simulink model "hybrid_photovoltaic_wind_power_sysytem_grid"  (R2024b)
settings: Solver=ode45  StartTime=0.0  StopTime=1  RelTol=1e-3  EnableMultiTasking=on
undefined symbols (not defined in the file): DiscIntNeverNeededParam, find_system
libraries: powerlib_extras x39, spsThreePhaseVIMeasurementLib x12, spsSeriesRLCBranchLib x5, spsDiodeLib x4, spsUniversalBridgeLib x4, simulink_extras x4, spsThreePhaseBreakerLib x3, spsLoadFlowBusLib x3, spsVoltageMeasurementLib x2, slpidlib x2, spsThreePhaseSeriesRLCLoadLib x2, spsThreePhaseTransformerInductanceMatrixTypeTwoWindingsLib x2
(part 1 of 4)
settings Model: Creator=venkat  LastModifiedBy=vinay
settings SolverCC: AlgebraicLoopSolver=TrustRegion
settings DataIOCC: LimitDataPoints=on  SaveFormat=Array  SignalLoggingSaveFormat=ModelDataLogs  ReturnWorkspaceOutputs=off
settings OptimizationCC: ExpressionDepthLimit=2147483647  LifeSpan=inf
settings DebuggingCC: UnderspecifiedInitializationDetection=Classic  MergeDetectMultiDrivingBlocksExec=none  SolverPrmCheckMsg=warning  FcnCallInpInsideContextMsg=warning  UnconnectedInputMsg=warning  UnconnectedOutputMsg=warning  UnconnectedLineMsg=warning  StateNameClashWarn=warning  SFUnexpectedBacktrackingDiag=warning  SFNoUnconditionalDefaultTransitionDiag=warning  SFExecutionAtInitializationDiag=none  ArithmeticOperatorsInVariantConditions=warning
settings HardwareCC: ProdBitPerPointer=32  ProdBitPerSizeT=32  ProdBitPerPtrDiffT=32  ProdLargestAtomicFloat=None  ProdIntDivRoundTo=Undefined  ProdEndianess=Unspecified  ProdWordSize=32  ProdHWDeviceType=32-bit Generic
settings ModelReferenceCC: EnableRefExpFcnMdlSchedulingChecks=on  PropagateSignalLabelsOutOfModel=off
settings SFSimCC: SimUseLocalCustomCode=off  CustomCodeUndefinedFunction=UseInterfaceOnly
settings RTWCC: RTWUseLocalCustomCode=off  GPUComputeCapability=3.5  DLArmComputeVersion=19.05
settings CodeAppCC: StateflowObjectComments=on
settings GRTTargetCC: TargetLangStandard=C89/C90 (ANSI)  CombineOutputUpdateFcns=off  GRTInterface=on
settings ConfigComp: CovMetricSettings=dw  CovSaveCumulativeToWorkspaceVar=on  CovSaveSingleToWorkspaceVar=on  CovExternalEMLEnable=off
settings SimscapeCC: SimscapeNormalizeSystem=off

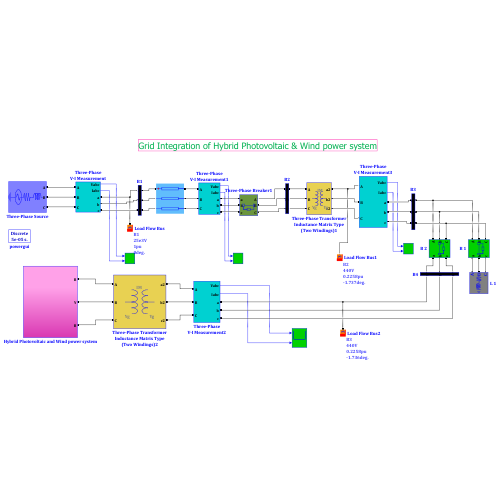
[thumbnail: Simulink's stored preview of the top-level diagram]
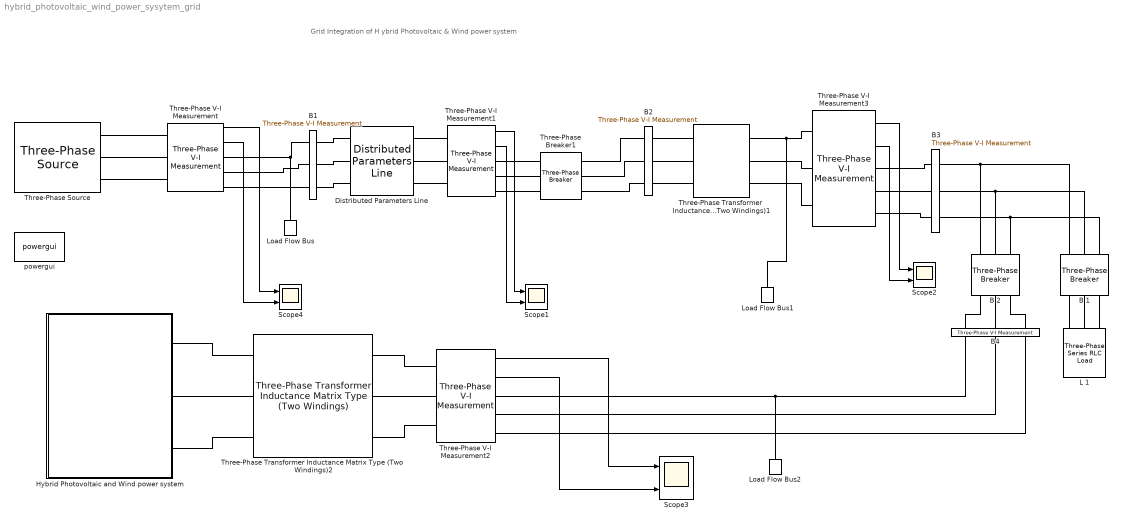
== system hybrid_photovoltaic_wind_power_sysytem_grid ==
  note: Grid Integration of H ybrid Photovoltaic & Wind power system
  B 1 : spsThreePhaseBreakerLib/Three-Phase Breaker  InitialState=closed  SwitchA=off  SwitchB=off  SwitchC=off  SwitchTimes="[0.02  0.4]"  External=off  BreakerResistance=0.001  SnubberResistance=1e6  SnubberCapacitance=inf  Measurements=None
  B 2 : spsThreePhaseBreakerLib/Three-Phase Breaker  InitialState=closed  SwitchA=off  SwitchB=off  SwitchC=off  SwitchTimes=[0.001 0.3]  External=off  BreakerResistance=0.001  SnubberResistance=1e6  SnubberCapacitance=inf  Measurements=None
  B1 : spsThreePhaseVIMeasurementLib/Three-Phase V-I Measurement  VoltageMeasurement=phase-to-ground  SetLabelV=on  LabelV=Vabc_B1  Vpu=off  VpuLL=off  CurrentMeasurement=no  SetLabelI=off  LabelI=A1  Ipu=off  Pbase=100e6  Vbase=25e3  OutputType=Magnitude  PhasorSimulation=off  PSBequivalent=0
  B2 : spsThreePhaseVIMeasurementLib/Three-Phase V-I Measurement  VoltageMeasurement=phase-to-ground  SetLabelV=on  LabelV=Vabc_B2  Vpu=off  VpuLL=off  CurrentMeasurement=yes  SetLabelI=on  LabelI=A2  Ipu=off  Pbase=100e6  Vbase=440  OutputType=Magnitude  PhasorSimulation=off  PSBequivalent=0
  B3 : spsThreePhaseVIMeasurementLib/Three-Phase V-I Measurement  VoltageMeasurement=phase-to-ground  SetLabelV=on  LabelV=Vabc_B3  Vpu=off  VpuLL=off  CurrentMeasurement=yes  SetLabelI=on  LabelI=A1  Ipu=off  Pbase=100e6  Vbase=440  OutputType=Magnitude  PhasorSimulation=off  PSBequivalent=0
  B4 : spsThreePhaseVIMeasurementLib/Three-Phase V-I Measurement  VoltageMeasurement=phase-to-phase  SetLabelV=on  LabelV=Vabc_B4  Vpu=off  VpuLL=off  CurrentMeasurement=yes  SetLabelI=on  LabelI=Iabc_B4  Ipu=off  Pbase=100e6  Vbase=440  OutputType=Magnitude  PhasorSimulation=off  PSBequivalent=0
  Distributed Parameters Line : spsDistributedParametersLineLib/Distributed Parameters Line  Phases=3  Length=100  Frequency=50  Resistance=[0.01273 0.3864]  Inductance="[0.9337e-3  4.1264e-3]"  Capacitance=[12.74e-9 7.751e-9]  x1=[-0.0006 7.90669957622914e-08 8343.04989423718 -24001.8540044251;-0.00055 7.82728037889709e-08 8719.02536979415 -23867.8460232251;-0.0005 7.74592991725365e-08 9092.84955630671 -23727.949008161;-0.00045 7.66266826330796e-08 9464.43021825048 -23582.1974767281;-0.0004 7.57751596062727e-08 9833.67567365721 -23430.6273909358;-0.00035 7.4904940192681e-08 10200.4948167359 -23273.2761484348;-0.0003 7.40162391059235e-08 10564.7971403519 -23110.1825732897;-0.00025 7.31092756196953e-08 10926.4927583579 -22941.3869063997;-0.0002 7.21842735136655e-08 11285.4924277724 -22766.9307955699;-0.00015 7.12414610182627e-08 11641.7075707988 -22586.8572852351;-0.0001 7.02810707583625e-08 11995.0502966807 -22401.2108058397;-5e-05 6.9303339695891e-08 12345.4334233877 -22210.0371628744]  x2=[-0.0006 3.59900680263241e-07 8376.65197170131 -24147.4259529429;-0.00055 3.57111090981103e-07 8754.90984663917 -24012.8722144004;-0.0005 3.54233389880834e-07 9131.0075785749 -23872.3936589513;-0.00045 3.51268286992119e-07 9504.85237102082 -23726.0249475771;-0.0004 3.4821651390973e-07 9876.35198336835 -23573.8021945673;-0.00035 3.45078823613009e-07 10245.414753647 -23415.7629586084;-0.0003 3.41855990280087e-07 10611.9496211406 -23251.946233517;-0.00025 3.38548809096864e-07 10975.8661488553 -23082.3924386188;-0.0002 3.35158096060811e-07 11337.0745458331 -22907.1434087756;-0.00015 3.31684687779633e-07 11695.485689307 -22726.2423840633;-0.0001 3.2812944126485e-07 12051.0111466903 -22539.7339991027;-5e-05 3.24493233720341e-07 12403.5631973964 -22347.6642720472]  x3=[-0.0006 1.55337357382061e-09 21.0108746560212 -91.3718539054767;-0.00055 1.57888274892892e-09 22.4434892992346 -91.0305571114422;-0.0005 1.60400235834426e-09 23.8705663472925 -90.6667998895599;-0.00045 1.62872620417889e-09 25.2917536902872 -90.2806719914813;-0.0004 1.65304818619379e-09 26.7067006715075 -89.8722686884876;-0.00035 1.67696230330383e-09 28.115058173958 -89.4416907479825;-0.0003 1.70046265505846e-09 29.5164787064987 -88.9890444086301;-0.00025 1.72354344309752e-09 30.9106164895831 -88.5144413541416;-0.0002 1.74619897258194e-09 32.2971275405743 -88.017998685719;-0.00015 1.7684236535988e-09 33.675669758617 -87.4998388931622;-0.0001 1.79021200254063e-09 35.0459030090467 -86.9600898246467;-5e-05 1.81155864345835e-09 36.4074892073121 -86.3988846551788]  x4=[-0.0006 -9.48429281222997e-10 30.9094555729155 -89.1998043499292;-0.00055 -9.77841104130026e-10 32.3067319811332 -88.7032953647736;-0.0005 -1.00701165937636e-09 33.6960371866506 -88.1849001687826;-0.00045 -1.03593374956399e-09 35.0770283991967 -87.6447466682139;-0.0004 -1.06460023859991e-09 36.4493648798542 -87.0829681378614;-0.00035 -1.09300405345692e-09 37.8127080251312 -86.4997031881712;-0.0003 -1.12113818591871e-09 39.1667214505066 -85.8950957310422;-0.00025 -1.14899569430908e-09 40.5110710734284 -85.2692949443175;-0.0002 -1.17656970520466e-09 41.845425195743 -84.6224552349772;-0.00015 -1.20385341513088e-09 43.169454585537 -83.9547362010405;-0.0001 -1.23084009224056e-09 44.4828325583705 -83.266302592188;-5e-05 -1.25752307797493e-09 45.7852350578811 -82.5573242691113]  x5=0.000565541566995743  V1=ones(3,3)  V2=ones(3,3)  I1=ones(3,3)  I2=ones(3,3)  nHarmo=1  Measurements=None  Decoupling=off  VsMag0=0  VrMag0=0  VsAngle0=0  VrAngle0=0  IsMag0=0  IrMag0=0  IsAngle0=0  IrAngle0=0
  Hybrid Photovoltaic and Wind power system : Subsystem
  L 1 : spsThreePhaseSeriesRLCLoadLib/Three-Phase Series RLC Load  LConnTagsString=A|B|C  Configuration=Y (grounded)  NominalVoltage=254.04  Vabc=[1e3 1e3 1e3]  Vabcp=[1e3 1e3 1e3]  NominalFrequency=50  UnbalancedPower=off  ActivePower=50e3  InductivePower=100  CapacitivePower=0  Pabc=[10e3 9e3 11e3]  QLabc=[100 90 110]  QCabc=[100 90 110]  Pabcp=[10e3 9e3 11e3]  QLabcp=[100 90 110]  QCabcp=[100 90 110]  Measurements=None  LoadType=constant Z
  Load Flow Bus : spsLoadFlowBusLib/Load Flow Bus  LConnTagsString=a  Phases=single  Connectors=on one side  ID=B1  Vbase=25e3  Vref=1  Vangle=0  VLF=1  VLFb=1  VLFc=1  angleLF=0  angleLFb=0  angleLFc=0
      settings: AttributesFormatString=%<ID>\n%<Vbase>V\n%<VLF>pu\n%<angleLF>deg.
  Load Flow Bus1 : spsLoadFlowBusLib/Load Flow Bus  LConnTagsString=a  Phases=single  Connectors=on one side  ID=B2  Vbase=440  Vref=1  Vangle=0  VLF=0.2258  VLFb=1  VLFc=1  angleLF=-1.737  angleLFb=0  angleLFc=0
      settings: AttributesFormatString=%<ID>\n%<Vbase>V\n%<VLF>pu\n%<angleLF>deg.
  Load Flow Bus2 : spsLoadFlowBusLib/Load Flow Bus  LConnTagsString=a  Phases=single  Connectors=on one side  ID=B3  Vbase=440  Vref=1  Vangle=0  VLF=0.2258  VLFb=1  VLFc=1  angleLF=-1.736  angleLFb=0  angleLFc=0
      settings: AttributesFormatString=%<ID>\n%<Vbase>V\n%<VLF>pu\n%<angleLF>deg.
  Scope{1..4} (4 alike) : Scope  NumInputPorts=2
  Three-Phase V-I Measurement{,1..3} (4 alike) : spsThreePhaseVIMeasurementLib/Three-Phase V-I Measurement  VoltageMeasurement=phase-to-ground  SetLabelV=off  LabelV=Vabc  Vpu=off  VpuLL=off  CurrentMeasurement=yes  SetLabelI=off  LabelI=Iabc  Ipu=off  Pbase=100e6  Vbase=500e3  OutputType=Complex  PhasorSimulation=off  PSBequivalent=0
  Three-Phase Breaker1 : spsThreePhaseBreakerLib/Three-Phase Breaker  InitialState=closed  SwitchA=off  SwitchB=off  SwitchC=off  SwitchTimes="[1/50  20/50]"  External=off  BreakerResistance=0.001  SnubberResistance=1e6  SnubberCapacitance=inf  Measurements=None
  Three-Phase Source : spsThreePhaseSourceLib/Three-Phase Source  InternalConnection=Yg  VoltagePhases=off  Voltage=(25000)*1.00008  PhaseAngle=0.13223  Voltage_phases=[25e3 25e3 25e3]/sqrt(3)  PhaseAngles_phases=[0 -120 +120]  Frequency=50  NonIdealSource=on  SpecifyImpedance=on  Resistance=0.8929  Inductance=16.58e-3  ShortCircuitLevel=100e6  BaseVoltage=63510.4  XRratio=7  BusType=swing  Pref=0  Qref=0  Prefabc=[10e3, 10e3, 10e3]  Qrefabc=[0, 0, 0]  Qmin=-inf  Qmax=inf
  Three-Phase Transformer Inductance Matrix Type (Two Windings)1 : spsThreePhaseTransformerInductanceMatrixTypeTwoWindingsLib/Three-Phase Transformer Inductance Matrix Type (Two Windings)  CoreType=Three-limb or five-limb core  Winding1Connection=Yg  Winding2Connection=Yg  AutoTransformer=off  Measurements=None  NominalPower=[100e3 50]  VLLnom=[63510.4 254.03]  WindingResistances=[0.01 0.01]  NoLoadIexcPos=2  NoLoadPlossPos=1000  ShortCircuitReactancePos=0.06  ShortCircuitReactancePosAuto=0.06  NoLoadIexcZero=100  NoLoadPlossZero=1500  ShortCircuitReactanceZero=0.03  ShortCircuitReactanceZeroAuto=0.03
  Three-Phase Transformer Inductance Matrix Type (Two Windings)2 : spsThreePhaseTransformerInductanceMatrixTypeTwoWindingsLib/Three-Phase Transformer Inductance Matrix Type (Two Windings)  CoreType=Three-limb or five-limb core  Winding1Connection=Yg  Winding2Connection=Yg  AutoTransformer=off  Measurements=None  NominalPower=[100e3 50]  VLLnom=[254.03 254.03]  WindingResistances=[0.01 0.01]  NoLoadIexcPos=2  NoLoadPlossPos=1000  ShortCircuitReactancePos=0.06  ShortCircuitReactancePosAuto=0.06  NoLoadIexcZero=100  NoLoadPlossZero=1500  ShortCircuitReactanceZero=0.03  ShortCircuitReactanceZeroAuto=0.03
  powergui : spspowerguiLib/powergui  Priority=1  SimulationMode=Discrete  SampleTime=50e-6  frequency=60  Iterations=50  frequencyindice=0  Pbase=100e6  ErrMax=0.0001  UnitsV=kV  UnitsW=MW  buscounter=0  FunctionMessages=off  echomessages=off  EnableUseOfTLC=off  CurrentSourceSwitches=off  DisableSnubberDevices=off  DisableRonSwitches=off  DisableVfSwitches=off  DisplayEquations=off  AutomaticDiscreteSolvers=off  SolverType=Tustin  Interpol=off  ExternalGateDelay=off  methode=off  Ts=100  x0status=blocks  SPID=off  SwTol=0  HookPort=off  NonlinearTolerance=1e-4  nMaxIteration=100  ContinueOnMaxIteration=off  RestoreLinks=warning  ResistiveCurrentMeasurement=off  Frange=[0:2:500]  Ylog=off  Xlog=on  ShowGrid=off  save=off  variable=ZData  structure=MLFCDSTAT  ZoomFFT=off  StartTime=0.8  cycles=10  DisplayStyle=1  fundamental=50  FreqAxis=on  MaxFrequency=50000  frequencyindicesteady=1  RmsSteady=1  display=off
  wires:
  Three-Phase V-I Measurement1/1 -> Scope1/1
  Three-Phase V-I Measurement1/2 -> Scope1/2
  Three-Phase V-I Measurement/1 -> Scope4/1
  Three-Phase V-I Measurement/2 -> Scope4/2
  Three-Phase V-I Measurement2/1 -> Scope3/1
  Three-Phase V-I Measurement2/2 -> Scope3/2
  Three-Phase V-I Measurement3/1 -> Scope2/1
  Three-Phase V-I Measurement3/2 -> Scope2/2
  connections:
  Three-Phase V-I Measurement/LConn3 -- Three-Phase Source/RConn3
  Three-Phase V-I Measurement/LConn2 -- Three-Phase Source/RConn2
  Three-Phase V-I Measurement/LConn1 -- Three-Phase Source/RConn1
  Three-Phase V-I Measurement/RConn3 -- B1/RConn3
  Three-Phase V-I Measurement/RConn2 -- B1/RConn2
  Three-Phase V-I Measurement/RConn1 -- Load Flow Bus/LConn1 -- B1/RConn1
  Distributed Parameters Line/LConn3 -- B1/LConn3
  Distributed Parameters Line/LConn2 -- B1/LConn2
  Distributed Parameters Line/LConn1 -- B1/LConn1
  Three-Phase V-I Measurement1/LConn3 -- Distributed Parameters Line/RConn3
  Three-Phase V-I Measurement1/LConn2 -- Distributed Parameters Line/RConn2
  Three-Phase V-I Measurement1/LConn1 -- Distributed Parameters Line/RConn1
  Three-Phase Transformer Inductance Matrix Type (Two Windings)1/LConn3 -- B2/LConn3
  Three-Phase Transformer Inductance Matrix Type (Two Windings)1/LConn2 -- B2/LConn2
  Three-Phase Transformer Inductance Matrix Type (Two Windings)1/LConn1 -- B2/LConn1
  Three-Phase V-I Measurement3/LConn3 -- Three-Phase Transformer Inductance Matrix Type (Two Windings)1/RConn3
  Three-Phase V-I Measurement3/LConn2 -- Three-Phase Transformer Inductance Matrix Type (Two Windings)1/RConn2
  Three-Phase V-I Measurement3/LConn1 -- Three-Phase Transformer Inductance Matrix Type (Two Windings)1/RConn1 -- Load Flow Bus1/LConn1
  Three-Phase V-I Measurement3/RConn1 -- B3/RConn1
  Three-Phase V-I Measurement3/RConn2 -- B3/RConn2
  Three-Phase V-I Measurement3/RConn3 -- B3/RConn3
  Three-Phase Breaker1/RConn1 -- Three-Phase V-I Measurement1/RConn1
  Three-Phase Breaker1/RConn2 -- Three-Phase V-I Measurement1/RConn2
  Three-Phase Breaker1/RConn3 -- Three-Phase V-I Measurement1/RConn3
  Three-Phase Breaker1/LConn1 -- B2/RConn1
  Three-Phase Breaker1/LConn2 -- B2/RConn2
  Three-Phase Breaker1/LConn3 -- B2/RConn3
  Three-Phase Transformer Inductance Matrix Type (Two Windings)2/RConn1 -- Three-Phase V-I Measurement2/LConn1
  Three-Phase Transformer Inductance Matrix Type (Two Windings)2/RConn2 -- Three-Phase V-I Measurement2/LConn2
  Three-Phase Transformer Inductance Matrix Type (Two Windings)2/RConn3 -- Three-Phase V-I Measurement2/LConn3
  B4/LConn1 -- B 2/RConn1
  B4/LConn2 -- B 2/RConn2
  B4/LConn3 -- B 2/RConn3
  B4/RConn3 -- Three-Phase V-I Measurement2/RConn3
  B4/RConn2 -- Three-Phase V-I Measurement2/RConn2
  Three-Phase V-I Measurement2/RConn1 -- B4/RConn1 -- Load Flow Bus2/LConn1
  B 1/LConn1 -- B3/LConn1 -- B 2/LConn1
  B 1/LConn2 -- B 2/LConn2 -- B3/LConn2
  L 1/LConn1 -- B 1/RConn1
  B 1/RConn2 -- L 1/LConn2
  L 1/LConn3 -- B 1/RConn3
  Hybrid Photovoltaic and Wind power system/RConn1 -- Three-Phase Transformer Inductance Matrix Type (Two Windings)2/LConn1
  Hybrid Photovoltaic and Wind power system/RConn2 -- Three-Phase Transformer Inductance Matrix Type (Two Windings)2/LConn2
  Hybrid Photovoltaic and Wind power system/RConn3 -- Three-Phase Transformer Inductance Matrix Type (Two Windings)2/LConn3
  B 1/LConn3 -- B 2/LConn3 -- B3/LConn3

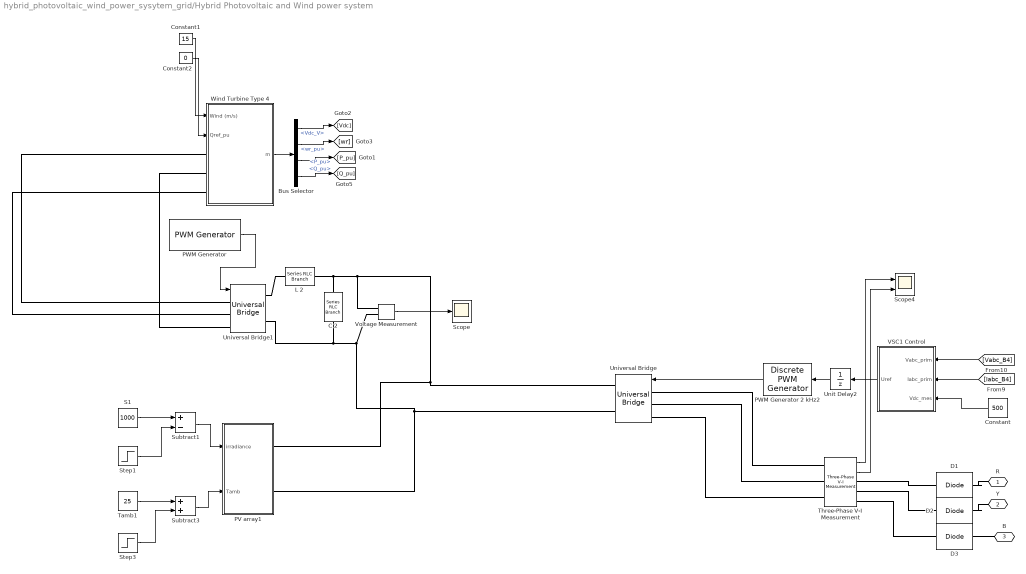
== system hybrid_photovoltaic_wind_power_sysytem_grid/Hybrid Photovoltaic and Wind power system ==
  Bus Selector : BusSelector  OutputSignals=Vdc_V,wr_pu,PQ_pu.P_pu,PQ_pu.Q_pu
  C 2 : spsSeriesRLCBranchLib/Series RLC Branch  LConnTagsString=__new0  RConnTagsString=__new0  BranchType=C  Resistance=1  Inductance=1e-4  SetiL0=off  InitialCurrent=0  Capacitance=3e-4  Setx0=off  InitialVoltage=0  Measurements=None
  Constant : Constant  Value=500
  Constant1 : Constant  Value=15
  Constant2 : Constant  Value=0
  D1 : spsDiodeLib/Diode  Ron=0.001  Lon=0  Vf=0.1  IC=0  UseSnubber=off  Rs=50000  Cs=250e-12  Measurements=off
  D2 : spsDiodeLib/Diode  Ron=0.001  Lon=0  Vf=0.1  IC=0  UseSnubber=off  Rs=50000  Cs=250e-12  Measurements=off
  D3 : spsDiodeLib/Diode  Ron=0.001  Lon=0  Vf=0.1  IC=0  UseSnubber=off  Rs=50000  Cs=250e-12  Measurements=off
  L 2 : spsSeriesRLCBranchLib/Series RLC Branch  LConnTagsString=__new0  RConnTagsString=__new0  BranchType=L  Resistance=1  Inductance=3e-2  SetiL0=off  InitialCurrent=0  Capacitance=1e-6  Setx0=off  InitialVoltage=0  Measurements=None
  PV array1 : Subsystem
  PWM Generator : powerlib_extras/Control  Blocks/PWM Generator  GeneratorMode="3-arm  bridge (6 pulses)"  Fc=1080  Internal=on  mIndex=0.4  Freq=50  Phase=0
  PWM Generator 2 kHz2 : powerlib_extras/Discrete  Control Blocks/Discrete PWM Generator  GeneratorMode="3-arm  bridge (6 pulses)"  Fc=33*50  Ts=1  Internal=off  mIndex=0.4  Freq=60  Phase=0
  S1 : Constant  Value=1000
  Scope : Scope
  Scope4 : Scope  NumInputPorts=2
  Step1 : Step  Time=3  After=200  SampleTime=0
  Step3 : Step  Time=2  After=5  SampleTime=0
  Subtract1 : Sum  Inputs=+-
  Subtract3 : Sum
  Tamb1 : Constant  Value=25
  Three-Phase V-I Measurement : spsThreePhaseVIMeasurementLib/Three-Phase V-I Measurement  VoltageMeasurement=phase-to-ground  SetLabelV=off  LabelV=Vabc  Vpu=off  VpuLL=off  CurrentMeasurement=yes  SetLabelI=off  LabelI=Iabc  Ipu=off  Pbase=100e6  Vbase=500e3  OutputType=Complex  PhasorSimulation=off  PSBequivalent=0
  Unit Delay2 : UnitDelay  HasFrameUpgradeWarning=on
  Universal Bridge : spsUniversalBridgeLib/Universal Bridge  Arms=3  SnubberResistance=1e5  SnubberCapacitance=inf  Device=MOSFET / Diodes  Ron=1e-3  Lon=0  ForwardVoltages="[  0  0  ]"  ForwardVoltage=0  GTOparameters=[ 10e-6 , 20e-6 ]  IGBTparameters=[ 1e-6 , 2e-6 ]  Measurements=None  Measurements_2=None  converterType=Rectifier
  Universal Bridge1 : spsUniversalBridgeLib/Universal Bridge  Arms=3  SnubberResistance=1e5  SnubberCapacitance=inf  Device=IGBT / Diodes  Ron=1e-3  Lon=0  ForwardVoltages="[  0  0  ]"  ForwardVoltage=0  GTOparameters=[ 10e-6 , 20e-6 ]  IGBTparameters=[ 1e-6 , 2e-6 ]  Measurements=None  Measurements_2=None  converterType=Rectifier
  VSC1 Control : Subsystem  mask(VSC Main Controller){nom=[ 50e3  50 ], Vnom=[ 6350.9 254.03 ], Vnom_dc=500, RLxfo=[0.008  0.04 ], RLchoke=[2e-3*(2*pi*60)/50   2e-3], K_VDCreg=[7  800], K_Ireg=[0.3 20]*1.5, Ts=1}
      mask prompts: nom "Nominal power and frequency [ Pnom(VA)  Fnom(Hz) ]:"; Vnom "Nominal primary and secondary voltages (Vrms LL) [ Vnom_prim   Vnom_sec ]:"; Vnom_dc "Nominal DC bus voltage (V):"; RLxfo "Total transformer leakage impedance (pu/Pnom) [ Rxfo  Lxf ]"; RLchoke "Choke impedance [ R(ohm) L(H) ]"; K_VDCreg "VDC regultator gains [ Kp  Ki ]:"; K_Ireg "Current regulator gains [ Kp  Ki ]:"; Ts "Sample time"
      mask init:
      | Pnom=nom(1);
      | Fnom=nom(2);
      | Vnom_prim=Vnom(1);
      | Vnom_sec=Vnom(2);
      | Zbase=Vnom_sec^2/Pnom;
      | Rtot_pu=RLxfo(1) + RLchoke(1)/Zbase;
      | Ltot_pu=RLxfo(2) + RLchoke(2)/(Zbase/(2*pi*Fnom));
      | Kp_VDCreg=K_VDCreg(1);
      | Ki_VDCreg=K_VDCreg(2);
      | Kp_Ireg=K_Ireg(1);
      | Ki_Ireg=K_Ireg(2);
      | Vdc_ref=Vnom_dc;
      | % Used to determine initial value of Boost Control (MPPT)
      | assignin('base','Vdc_ref_Inv',Vdc_ref);
  Voltage Measurement : spsVoltageMeasurementLib/Voltage Measurement  PhasorSimulation=off  OutputType=Complex  PSBequivalent=0
  Wind Turbine Type 4 : Subsystem  LoadFcn=%find_system(gcs,'FollowLinks', 'on', 'LookUnderMasks', 'all');  mask(Wind Turbine: Model 7){Nb_wt=1, ShowParameters=Control parameters for 1 wind turbine, nom=[1500/0.9 440 50], Reactances=[ 1.305, 0.296, 0.252, 0.474,  0.243,  0.18 ], Time_constants=[  4.49  0.0681  0.0513  ], Resistance=0.006, mec=[0.62 0.01 1], init=[ 0  0  0  0  0  0  0  0  1 ], Vnom=575, Imax_grid_conv=1.1, RL_grid=[ 0.15 0.15/50], C_var_filter1=150e3, Vdc_nom=1100, C_DClink1=90000e-6, L_R_Boost=[0.0012     5e-3], Pmec1=2e6, wind_speed_CpMax=11, wind0=11, DisplayTurbChar=off, H_WT=4.32, Ksh=0.3, D_mutual=1.5, w_wt0=1, torque0=1, Kdc=[1.1   27.5], Ki_var_reg=0.05, Ki_volt_reg=2, Kgrid_side_cur_reg=[1  50], Kspeed=[5 1], Kboost_cur_reg=[0.025 100], Kp_pitch=15, Kcompensation=[1.5  6], Kfield=[10  20], pitch_max=27, pitch_rate=10, Ts=0.1}
      mask prompts: Nb_wt "Number of wind turbines:"; ShowParameters "Display:"; nom "Nom. power, L-L volt. and freq.: [Pn (VA), Vn (Vrms), fn (Hz)]"; Reactances "Reactances [Xd Xd' Xd'' Xq Xq'' Xl] (p.u.):"; Time_constants "Time constants [Tdo' Tdo'' Tq''] (s):"; Resistance "Resistance Rs (p.u.):"; mec "Inertia constant, friction factor, and pairs of poles: [ H(s)  F(p.u.)  p ]"; init "Initial conditions: [dw(%) th(deg) ia,ib,ic(pu) pha,phb,phc(deg) Vf(pu)]:"; Vnom "Grid-side converter nominal AC voltage (V):"; Imax_grid_conv "Grid-side converter maximum AC current (pu based on generator power and converter nominal AC voltage):"; RL_grid "Grid-side coupling inductor [ L(pu) R(pu),pu based on generator power and converter nominal AC voltage] :"; C_var_filter1 "Line filter capacitor (Q=50) (var):"; Vdc_nom "Nominal DC bus voltage (V)"; C_DClink1 "DC bus capacitor (F):"; L_R_Boost "Boost converter inductance [L(H) R(ohm)]:"; Pmec1 "Nominal mechanical output power (W):"; wind_speed_CpMax "Wind speed at nominal speed and at Cp max (must be between 6 m/s and 30 m/s) (m/s):"; wind0 "Initial wind speed (m/s):"; DisplayTurbChar "Display wind turbine power characteristics:"; H_WT "Wind turbine inertia constant H (s):"; Ksh "Shaft spring constant refer to high-speed shaft (pu of nominal mechanical torque/rad):"; D_mutual "Shaft mutual damping (pu of nominal mechanical torque/pu dw):"; w_wt0 "Turbine initial speed (pu of nominal speed):"; torque0 "Initial output torque (pu of nominal mechanical torque):"; Kdc "DC bus voltage regulator gains [Kp Ki]:"; Ki_var_reg "Grid-side converter var regulator gain [ Ki]:"; Ki_volt_reg "Grid-side converter voltage regulator gain [ Ki]:"; Kgrid_side_cur_reg "Grid-side converter current regulator gains [Kp Ki]:"; Kspeed "Speed regulator gains [Kp Ki]:"; Kboost_cur_reg "Boost inductor current regulator gains [Kp Ki]:"; Kp_pitch "Pitch controller gain [Kp]:"; Kcompensation "Pitch compensation gains [Kp Ki]:"; Kfield "Field excitation gains [Kp Ki]:"; pitch_max "Maximum pitch angle (deg):"; pitch_rate "Maximum rate of change of pitch angle (deg/s)"; Ts "Sample time (s):"
      mask help: This block implements a model of a variable speed pitch controlled wind turbine using a synchronous generator.
      mask init:
      | %Generator data
      | Pnom=nom(1)*Nb_wt;
      | Vnom_gen=nom(2);
      | Fnom=nom(3);
      | Xd=Reactances(1);
      | Xd1=Reactances(2);
      | Xd2=Reactances(3);
      | Xq=Reactances(4);
      | Xq2=Reactances(5);
      | Xl=Reactances(6);
      | Tdo1=Time_constants(1);
      | Tdo2=Time_constants(2);
      | Tq2=Time_constants(3);
      | H=mec(1);
      | F=mec(2);
      | p=mec(3);
      | 
      | % Converters data
      | L_RL=RL_grid(1);
      | R_RL=RL_grid(2);
      | L_Boost=L_R_Boost(1)/Nb_wt;
      | R_Boost=L_R_Boost(2)/Nb_wt;
      | Q_filter=50;
      | C_DClink=C_DClink1*Nb_wt;
      | C_var_filter=C_var_filter1*Nb_wt;
      | 
      | % Controller data
      | Freq_filter=10000;   %Hz
      | Zeta_filter=0.707;
      | Kp_dc=Kdc(1);
      | Ki_dc=Kdc(2);
      | Kp_grid_side_cur_reg=Kgrid_side_cur_reg(1);
      | Ki_grid_side_cur_reg=Kgrid_side_cur_reg(2);
      | Kp_speed=Kspeed(1);
      | Ki_speed=Kspeed(2);
      | Kp_boost_cur_reg=Kboost_cur_reg(1);
      | Ki_boost_cur_reg=Kboost_cur_reg(2);
      | Kp_compensation=Kcompensation(1);
      | Ki_compensation=Kcompensation(2);
      | Kp_field=Kfield(1);
      | Ki_field=Kfield(2);
      | Mod_index_max=1.1;
      | T_speed=5;      %Speed reference time constant (s)
      | Iq_ref_limit_time_constant=0.3; %(s)
      | Current_reg_output_limit=1.1;   %(pu)
      | Var_reg_output_hi_limit=1.1;    %(pu)
      | Var_reg_output_low_limit=0.9;   %(pu)
      | Pitch_time_constant=0.01;       %(s)
      | Vf_limit=10;    %Field voltage limit (pu)
      | Flux_meas_time_constant=1*(1/Fnom); %(s)
      | Freq_sawtooth=2000; %Hz, Boost converter
      | Freq_PWM=3000; %Hz, Inverter
      | Ts_snub=50e-6;  %Sample time to compute snubber resistance
      | 
      | 
      | % Turbine data
      | Pmec=Pmec1*Nb_wt;
      | c1 = 0.6450;
      | c2 = 116;
      | c3 = .4;
      | c4 = 5;
      | c5 = 21;
      | c6 = .00912;  % Set Pmin in stall condition (does not vary with wind_speed_Pmax)
      | c7 = .08;
      | c8 = .035;
      | theta=0;
      | CpMax=.5;
      | lambda_CpMax=9.9495;
      | 
      | c1_c8=[c1 c2 c3 c4 c5 c6 c7 c8];
      |   
      | 
      | %   Cp = c1*(c6*lambda + (-c4 - c3*(2.5 + theta) + c2*(1/(lambda + ...
      | %   c7*(2.5 + theta)) - c8/(1 + (2.5 + theta)^3)))/exp(c5*(1/(lambda + ...
      | %   c7*(2.5 + theta)) - c8/(1 + (2.5 + theta)^3))))
      | 
      | 
      |         %%%%%%%%%%%%%%%%%%%%%%%%%%%%%%%%%%%%%%%%%%%%%%%%%%%%%%%%%%%%%%%%%%%%%%%%%%%
      |         % Operation at Cp max
      |         %%%%%%%%%%%%%%%%%%%%%%%%%%%%%%%%%%%%%%%%%%%%%%%%%%%%%%%%%%%%%%%%%%%%%%%%%%%
      |         
      |         rated_omegar=1;
      |         omegar = rated_omegar;
      |         
      |         % Enforce boundaries on wind speed
      |         % A warning could be displayed
      |         if wind_speed_CpMax < 6
      |             wind_speed_CpMax=6;
      |             disp('Warning: Wind speed at nominal speed and at Cp max has been set to 6 m/s')
      |         end
      |         if wind_speed_CpMax > 30
      |             wind_speed_CpMax=30;
      |             disp('Warning: Wind speed at nominal speed and at Cp max has been set to 30 m/s')
      |         end
      | 
      |         K1=lambda_CpMax/omegar*wind_speed_CpMax;
      |         
      |         % Calculation of K2 needed to get P equal to the requested value at
      |         % Cp max for the requested wind speed
      |         
      |         Prated=Pmec;
      |         P_rated_omegar_theta_zero=0.75;
      |         
      |         K2 = P_rated_omegar_theta_zero*Prated/(wind_speed_CpMax^3*CpMax);
      |         
      |         K1_K2=[K1 K2];
      |         
      |         %%%%%%%%%%%%%%%%%%%%%%%%%%%%%%%%%%%%%%%%%%%%%%%%%%%%%%%%%%%%%%%%%%%%%%%%%%%
      |         % End of calculation for operation at Cp max
      |         %%%%%%%%%%%%%%%%%%%%%%%%%%%%%%%%%%%%%%%%%%%%%%%%%%%%%%%%%%%%%%%%%%%%%%%%%%%
      |         
      | 
      | %%%%%%%%%%%%%%%%%%%%%%%%%%%%%%%%%%%%%%%%%%%%%%%%%%%%%%%%%%%%%%%%%%%%%%%%%%%
      | % Plot turbine characteristics
      | %%%%%%%%%%%%%%%%%%%%%%%%%%%%%%%%%%%%%%%%%%%%%%%%%%%%%%%%%%%%%%%%%%%%%%%%%%% 
      | 
      | DisplayTurbChar=get_param(gcb,'DisplayTurbChar');
      | if strcmp(DisplayTurbChar,'on')
      |     vect_theta = 0:2:30;
      |     
      |     vect_lambda = 1:0.2:30;
      |     
      |     clear Cp;
      |     
      |     for i=1:length(vect_theta)
      |      for j=1:length(vect_lambda)
      |                 Cp(i,j) = c1*(c6*vect_lambda(j) + (-c4 - c3*(2.5 + vect_theta(i)) + c2*(1/(vect_lambda(j) + ...
      |                 c7*(2.5 + vect_theta(i))) - c8/(1 + (2.5 + vect_theta(i))^3)))/exp(c5*(1/(vect_lambda(j) + ...
      |                 c7*(2.5 + vect_theta(i))) - c8/(1 + (2.5 + vect_theta(i))^3))));
      |      end
      |     end
      | 
      |     figure(1);
      |     clf;
      |     hold on;
      | 
      |     plot(vect_lambda, Cp);
      |     axis([0, 25, 0, .6]);
      |     title('Wind Turbine Cp Characteristic (pitch angle increases by step of 2 deg.)');
      |     ylabel('Cp');
      |     set(gca,'ytick',[0 .1 .2 .3 .4 .5 .6]);
      |     xlabel('Lambda');
      |     grid on;
      |     text(10.1,0.51,'Pitch angle 0 degree');
      | 
      |     hold off
      |     
      |     % Plot of the wind turbine mechanical power output (pu) lambda and Cp
      |     % characteristics against wind speed (m/s) for a range of theta.
      |     
      |     wind_speed_range = [1,.2,30];
      |     vect_wind_speed = 1:0.2:30;
      |     
      |     clear lambda;
      |     clear Cp;
      |     clear P;
      | 
      |     for i=1:length(vect_theta)
      |         for j=1:length(vect_wind_speed)
      |             lambda(i,j) = K1*omegar/vect_wind_speed(j);
      |             Cp(i,j) = c1*(c6*lambda(i,j) + (-c4 - c3*(2.5 + vect_theta(i)) + c2*(1/(lambda(i,j) + ...
      |             c7*(2.5 + vect_theta(i))) - c8/(1 + (2.5 + vect_theta(i))^3)))/exp(c5*(1/(lambda(i,j) + ...
      |             c7*(2.5 + vect_theta(i))) - c8/(1 + (2.5 + vect_theta(i))^3))));
      |             P(i,j) = K2/Prated*vect_wind_speed(j)^3*Cp(i,j);
      |         end
      |     end
      |     
      |     
      |     figure(2);
      |     clf;
      |     hold on
      |     
      |     subplot(3,1,1);
      |     plot(vect_wind_speed, P);
      |     axis([0, 35, 0, 1.5]);
      |     title('Wind Turbine Characteristics (w = 1 pu, pitch angle increases by step of 2 deg.)');
      |     ylabel('P (pu)');
      |     set(gca,'ytick',0:.5:4);
      |     grid on;
      |     
      |     subplot(3,1,2);
      |     plot(vect_wind_speed, lambda);
      |     axis([0, 35, 0, 20]);
      |     ylabel('Lambda');
      |     grid on;
      |     
      |     subplot(3,1,3)
      |     plot(vect_wind_speed, Cp);
      |     axis([0, 35, 0, .6]);
      |     xlabel('Wind Speed (m/s)');
      |     ylabel('Cp');
      |     set(gca,'ytick',[0 .1 .2 .3 .4 .5 .6]);
      |     grid on;
      | 
      |     hold off
      |     set_param(gcb,'DisplayTurbChar','off')
      |     
      | end
      mask TypeOptions ShowParameters: Generator data for 1 wind turbine | Converters data for 1 wind turbine | Turbine data for 1 wind turbine | Drive train data for 1 wind turbine | Control parameters for 1 wind turbine
      mask Callback ShowParameters:
      | BlockName=getfullname(gcb);
      | %
      | Param_Show=get_param(BlockName,'ShowParameters');
      | Param_DisplayTurbChar=get_param(BlockName,'DisplayTurbChar');
      | 
      | p_mask{3}='off';p_mask{4}='off';p_mask{5}='off';
      | p_mask{6}='off';p_mask{7}='off';p_mask{8}='off';p_mask{9}='off';
      | p_mask{10}='off';p_mask{11}='off';p_mask{12}='off';p_mask{13}='off';
      | p_mask{14}='off';p_mask{15}='off';p_mask{16}='off';p_mask{17}='off';
      | p_mask{18}='off';p_mask{19}='off';p_mask{20}='off';p_mask{21}='off';
      | p_mask{22}='off';p_mask{23}='off';p_mask{24}='off';p_mask{25}='off';
      | p_mask{26}='off';p_mask{27}='off';p_mask{28}='off';p_mask{29}='off';
      | p_mask{30}='off';p_mask{31}='off';p_mask{32}='off';p_mask{33}='off';
      | p_mask{34}='off';p_mask{35}='off';
      | 
      | switch Param_Show
      | 	case 'Generator data for 1 wind turbine'
      | 		p_mask{3}='on';p_mask{4}='on';p_mask{5}='on';
      |         p_mask{6}='on';p_mask{7}='on';p_mask{8}='on';
      |     case 'Converters data for 1 wind turbine'
      | 		p_mask{9}='on';p_mask{10}='on';p_mask{11}='on';
      |         p_mask{12}='on';p_mask{13}='on';p_mask{14}='on';p_mask{15}='on';
      | 	case 'Turbine data for 1 wind turbine'
      | 		p_mask{16}='on';p_mask{17}='on';p_mask{18}='on';p_mask{19}='on';
      |     case 'Drive train data for 1 wind turbine'
      |         p_mask{20}='on';p_mask{21}='on';p_mask{22}='on';p_mask{23}='on';
      |         p_mask{24}='on';
      |     case 'Control parameters for 1 wind turbine'
      |         p_mask{25}='on';p_mask{26}='on';p_mask{27}='on';
      |         p_mask{28}='on';p_mask{29}='on';p_mask{30}='on';p_mask{31}='on';
      |         p_mask{32}='on';p_mask{33}='on';p_mask{34}='on';p_mask{35}='on';
      | end
      | 
      | ParVisible={'on','on',p_mask{3},p_mask{4},p_mask{5},p_mask{6},...
      |     p_mask{7},p_mask{8},p_mask{9},p_mask{10},p_mask{11},p_mask{12},...
      |     p_mask{13},p_mask{14},p_mask{15},p_mask{16},p_mask{17},p_mask{18},...
      |     p_mask{19},p_mask{20},p_mask{21},p_mask{22},p_mask{23},p_mask{24},...
      |     p_mask{25},p_mask{26},p_mask{27},p_mask{28},p_mask{29},p_mask{30},...
      |     p_mask{31},p_mask{32},p_mask{33},p_mask{34},p_mask{35},'on'};
      | %
      | set_param(BlockName,'MaskVisibilities',ParVisible);
      | set_param(BlockName,'DisplayTurbChar',Param_DisplayTurbChar);
      mask Display: disp(' ');
  R : PMIOPort  Side=Right
  Y : PMIOPort  Port=2  Side=Right
  B : PMIOPort  Port=3  Side=Right
  wires:
  [Vabc_B4] -> VSC1 Control/1(Vabc_prim)
  [Iabc_B4] -> VSC1 Control/2(Iabc_prim)
  PWM Generator 2 kHz2/1 -> Universal Bridge/1
  Constant/1 -> VSC1 Control/3(Vdc_mes)
  Three-Phase V-I Measurement/1 -> Scope4/1
  Three-Phase V-I Measurement/2 -> Scope4/2
  Unit Delay2/1 -> PWM Generator 2 kHz2/1
  VSC1 Control/1(Uref) -> Unit Delay2/1
  Voltage Measurement/1 -> Scope/1
  Subtract3/1 -> PV array1/2(Tamb)
  S1/1 -> Subtract1/1
  Subtract1/1 -> PV array1/1(irradiance)
  Step1/1 -> Subtract1/2
  Tamb1/1 -> Subtract3/1
  Step3/1 -> Subtract3/2
  Constant1/1 -> Wind Turbine Type 4/1("Wind (m/s) ")
  Wind Turbine Type 4/1(m) -> Bus Selector/1
  Constant2/1 -> Wind Turbine Type 4/2(Qref_pu)
  Bus Selector/1 -> [Vdc]  "<Vdc_V>"
  Bus Selector/2 -> [wr]  "<wr_pu>"
  Bus Selector/3 -> [P_pu]  "<P_pu>"
  Bus Selector/4 -> [Q_pu]  "<Q_pu>"
  PWM Generator/1 -> Universal Bridge1/1
  connections:
  Three-Phase V-I Measurement/LConn1 -- Universal Bridge/LConn1
  Three-Phase V-I Measurement/LConn2 -- Universal Bridge/LConn2
  Three-Phase V-I Measurement/RConn2 -- D2/LConn1
  D3/RConn1 -- B/RConn1
  D2/RConn1 -- Y/RConn1
  Three-Phase V-I Measurement/LConn3 -- Universal Bridge/LConn3
  Three-Phase V-I Measurement/RConn1 -- D1/LConn1
  D1/RConn1 -- R/RConn1
  Three-Phase V-I Measurement/RConn3 -- D3/LConn1
  Voltage Measurement/LConn1 -- PV array1/RConn1 -- Universal Bridge/RConn1 -- C 2/LConn1 -- L 2/RConn1
  PV array1/RConn2 -- Voltage Measurement/LConn2 -- Universal Bridge1/RConn2 -- C 2/RConn1 -- Universal Bridge/RConn2
  L 2/LConn1 -- Universal Bridge1/RConn1
  Wind Turbine Type 4/LConn3 -- Universal Bridge1/LConn2
  Wind Turbine Type 4/LConn1 -- Universal Bridge1/LConn1
  Wind Turbine Type 4/LConn2 -- Universal Bridge1/LConn3

== system hybrid_photovoltaic_wind_power_sysytem_grid/Hybrid Photovoltaic and Wind power system/PV array1 ==
  irradiance : Inport
  Tamb : Inport  Port=2
  4700uF : spsSeriesRLCBranchLib/Series RLC Branch  LConnTagsString=__new0  RConnTagsString=__new0  BranchType=C  Resistance=1  Inductance=5e-03  SetiL0=off  InitialCurrent=0  Capacitance=4700e-6  Setx0=off  InitialVoltage=0  Measurements=None
  CCS : spsControlledCurrentSourceLib/Controlled Current Source  Initialize=on  Source_Type=AC  Amplitude=0  Phase=0  Frequency=0  Measurements=None
  CM : spsCurrentMeasurementLib/Current Measurement  PhasorSimulation=off  OutputType=Complex  PSBequivalent=0
  Divide1 : Product  Inputs=**
  Im : Constant  Value=1.93
  Isc : Constant  Value=2.02
  Saturation : Saturate  UpperLimit=100  LowerLimit=0
  Saturation1 : Saturate  UpperLimit=4  LowerLimit=0
  Subsystem1 : Subsystem
  Tref : Constant  Value=55
  VM1 : spsVoltageMeasurementLib/Voltage Measurement  PhasorSimulation=off  OutputType=Complex  PSBequivalent=0
  Vm : Constant  Value=70.4
  Voc : Constant  Value=86.8
  + : PMIOPort  Tag=PMCPort  Side=Right
  - : PMIOPort  Tag=PMCPort  Port=2  Side=Right
  tag scope: Ipv1=global, Ppv1=global, Upv1=global
  wires:
  Saturation1/1 -> CCS/1
  CM/1 -> Divide1/2, [Ipv1]
  Divide1/1 -> [Ppv1]
  Subsystem1/2(Ipv) -> Saturation1/1
  Tref/1 -> Subsystem1/9(Tref)
  VM1/1 -> Divide1/1, [Upv1], Saturation/1
  Saturation/1 -> Subsystem1/1(Vpv)
  Tamb/1 -> Subsystem1/3(Tamb)
  irradiance/1 -> Subsystem1/2(S)
  Vm/1 -> Subsystem1/8(Vm)
  Voc/1 -> Subsystem1/6(Voc)
  Im/1 -> Subsystem1/7(Im)
  Isc/1 -> Subsystem1/4(Isc)
  Subsystem1/1(Out1) -> Subsystem1/5(In5)
  connections:
  4700uF/RConn1 -- VM1/LConn2 -- CCS/LConn1 -- -/RConn1
  4700uF/LConn1 -- VM1/LConn1 -- CM/RConn1 -- +/RConn1
  CCS/RConn1 -- CM/LConn1

== system hybrid_photovoltaic_wind_power_sysytem_grid/Hybrid Photovoltaic and Wind power system/VSC1 Control ==
  note: VSC Main Controller
  Vabc_prim : Inport  PortDimensions=3
  Iabc_prim : Inport  Port=2  PortDimensions=3
  Vdc_mes : Inport  Port=3  PortDimensions=1
  Current Regulator : Subsystem
  Gain : Gain  Gain=-1
  Iq_ref : Constant  Value=0
  Mux : Mux  Inputs=2
  PLL & Measurements : Subsystem
  Uabc_ref Generation max (m) = 1 : Subsystem
  VDC Regulator : Subsystem
  Vdc_ref1 : Constant  Value=Vdc_ref
  Uref : Outport
  wires:
  Vdc_ref1/1 -> VDC Regulator/2(Vdc_ref)
  Uabc_ref Generation max (m) = 1/1(Uabc_ref) -> Uref/1
  Iabc_prim/1 -> Gain/1
  Vabc_prim/1 -> PLL & Measurements/1(Vabc_prim)
  Vdc_mes/1 -> VDC Regulator/1(Vdc_mes)
  PLL & Measurements/2(VdVq_prim) -> Current Regulator/1(VdVq_mes)
  PLL & Measurements/3(IdIq_prim) -> Current Regulator/2(IdIq_mes)
  Mux/1 -> Current Regulator/3(IdIq_ref)
  Iq_ref/1 -> Mux/2
  Current Regulator/1(VdVq_conv) -> Uabc_ref Generation max (m) = 1/2(VdVq_conv)
  PLL & Measurements/1(wt) -> Uabc_ref Generation max (m) = 1/1(wt)
  VDC Regulator/1(Id_ref) -> Mux/1
  Gain/1 -> PLL & Measurements/2(Iabc_prim)

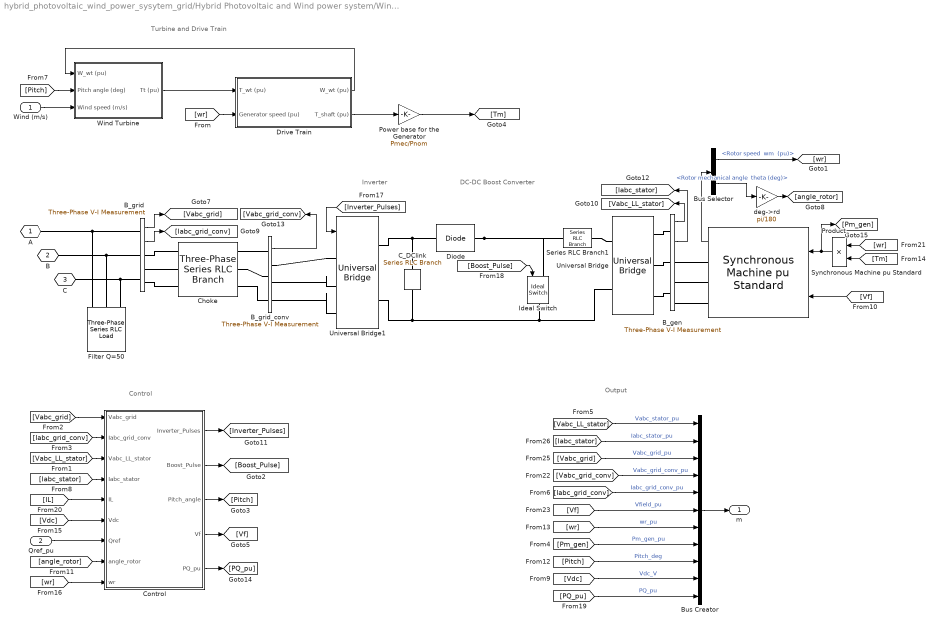
== system hybrid_photovoltaic_wind_power_sysytem_grid/Hybrid Photovoltaic and Wind power system/Wind Turbine Type 4 ==
  note: Turbine and Drive Train
  note: Control
  note: Inverter
  note: DC-DC Boost Converter
  note: Output
  "Wind (m/s) " : Inport
  Qref_pu : Inport  Port=2
  B_gen : spsThreePhaseVIMeasurementLib/Three-Phase V-I Measurement  VoltageMeasurement=phase-to-phase  SetLabelV=off  LabelV=Vabc  Vpu=on  VpuLL=off  CurrentMeasurement=yes  SetLabelI=off  LabelI=Iabc  Ipu=on  Pbase=Pnom  Vbase=Vnom_gen  OutputType=Complex  PhasorSimulation=off  PSBequivalent=0
  B_grid : spsThreePhaseVIMeasurementLib/Three-Phase V-I Measurement  VoltageMeasurement=phase-to-ground  SetLabelV=off  LabelV=Vabc  Vpu=on  VpuLL=off  CurrentMeasurement=yes  SetLabelI=off  LabelI=Iabc  Ipu=on  Pbase=Pnom  Vbase=Vnom  OutputType=Complex  PhasorSimulation=off  PSBequivalent=0
  B_grid_conv : spsThreePhaseVIMeasurementLib/Three-Phase V-I Measurement  VoltageMeasurement=phase-to-ground  SetLabelV=off  LabelV=Vabc  Vpu=on  VpuLL=off  CurrentMeasurement=no  SetLabelI=off  LabelI=Iabc  Ipu=on  Pbase=Pnom  Vbase=Vnom  OutputType=Complex  PhasorSimulation=off  PSBequivalent=0
  Bus Creator : BusCreator  Inputs=11
  Bus Selector : BusSelector  OutputSignals="Mechanical.Rotor speed  wm  (pu),Mechanical.Rotor mechanical angle  theta (deg)"
  C_DClink : spsSeriesRLCBranchLib/Series RLC Branch  LConnTagsString=__new0  RConnTagsString=__new0  BranchType=C  Resistance=1  Inductance=1e-3  SetiL0=off  InitialCurrent=0  Capacitance=C_DClink  Setx0=on  InitialVoltage=Vdc_nom  Measurements=Branch voltage
  "Choke " : spsThreePhaseSeriesRLCBranchLib/Three-Phase Series RLC Branch  LConnTagsString=A|B|C  RConnTagsString=A|B|C  BranchType=RL  Resistance=R_RL*Vnom^2/Pnom  Inductance=L_RL*Vnom^2/Pnom/(2*pi*Fnom)  Capacitance=[]  Measurements=None
  Control : Subsystem
  Diode : spsDiodeLib/Diode  Ron=1e-6/Nb_wt  Lon=0  Vf=0  IC=0  UseSnubber=off  Rs=inf  Cs=inf  Measurements=off
  Drive Train : Subsystem  mask(Wind Turbine shaft){H_WT=H_WT, Ksh=Ksh, D_mutual=D_mutual, wbase=2*pi*Fnom/p, w_wt0=w_wt0, torque0=torque0, Ts=Ts}
      mask prompts: H_WT "Wind turbine inertia constant H (s):"; Ksh "Shaft spring constant (pu of nominal mechanical torque/rad):"; D_mutual "Shaft mutual damping (pu of nominal mechanical torque/pu dw):"; wbase "Shaft base speed (rad/s):"; w_wt0 "Turbine initial speed (pu of base speed):"; torque0 "Initial output torque (pu of nominal mechanical torque):"; Ts "Sample time (s):"
      mask help:
      | This block implements a wind turbine drive train model. All shaft parameters are referred to high-speed shaft (generator shaft).
      |
      | The first input is the wind turbine torque in per unit (pu) based on the nominal power of the turbine and the base speed of the generator. The second input is the generator speed in pu based on the base speed of the generator.
      |
      | The outputs are:
      | 1- the transmitted torque of the shaft in pu based on the nominal power of the turbine and the base speed of the generator.
      | 2- the wind turbine speed in pu of the base speed of the generator.
  Filter Q=50 : spsThreePhaseSeriesRLCLoadLib/Three-Phase Series RLC Load  LConnTagsString=A|B|C  Configuration=Y (grounded)  NominalVoltage=Vnom  Vabc=[1e3 1e3 1e3]  Vabcp=[1e3 1e3 1e3]  NominalFrequency=Fnom  UnbalancedPower=off  ActivePower=C_var_filter/Q_filter  InductivePower=0  CapacitivePower=C_var_filter  Pabc=[10e3 9e3 11e3]  QLabc=[100 90 110]  QCabc=[100 90 110]  Pabcp=[10e3 9e3 11e3]  QLabcp=[100 90 110]  QCabcp=[100 90 110]  Measurements=None  LoadType=constant Z
  Ideal Switch : spsIdealSwitchLib/Ideal Switch  Ron=1e-6/Nb_wt  Lon=0  IC=0  Rs=1e5/Nb_wt  Cs=inf  Measurements=off
  Power base for the Generator : Gain  Gain=Pmec/Pnom  SaturateOnIntegerOverflow=on  OutDataTypeStr=Inherit: Same as input  ParamDataTypeStr=Inherit: Same as input
  Product : Product  RndMeth=Zero
  Series RLC Branch1 : spsSeriesRLCBranchLib/Series RLC Branch  LConnTagsString=__new0  RConnTagsString=__new0  BranchType=RL  Resistance=R_Boost  Inductance=L_Boost  SetiL0=off  InitialCurrent=0  Capacitance=1.0  Setx0=off  InitialVoltage=0  Measurements=Branch current
  Synchronous Machine pu Standard : spsSynchronousMachinepuStandardLib/Synchronous Machine pu Standard  PresetModel=No  MechanicalLoad=Mechanical power Pm  ShowDetailedParameters=on  RotorType=Salient-pole  Units=per unit standard parameters  MeasurementBus=off  NominalParameters="[ Pnom  Vnom_gen Fnom ]"  Reactances1=[ 1.81, 0.3, 0.23, 1.76, 0.65, 0.25, 0.15 ]  Reactances2="[ Xd, Xd1, Xd2, Xq,  Xq2,  Xl ]"  dAxisTimeConstants=Open-circuit  qAxisTimeConstants=Short-circuit  TimeConstants1="[ 4.4849  0.0681  0.1  ]"  TimeConstants2=[ 8.0, 0.03, 1.0, 0.07 ]  TimeConstants3="[  Tdo1  Tdo2  Tq2  ]"  TimeConstants4=[ 8.0, 0.03, 0.3371, 0.0295 ]  TimeConstants5=[ 1.01, 0.053, 0.1 ]  TimeConstants6=[ 1.3201, 0.023, 1.0, 0.07 ]  TimeConstants7="[  1.01  0.053  0.051266  ]"  TimeConstants8=[ 1.3201, 0.0231, 0.3371, 0.0295 ]  StatorResistance=Resistance  Mechanical=[ H F p]  PolePairs=1  InitialConditions=init  SetSaturation=off  Saturation=[0.6404,0.7127,0.8441,0.9214,0.9956,1.082,1.19,1.316,1.457;0.7,0.7698,0.8872,0.9466,0.9969,1.046,1.1,1.151,1.201]  LoadFlowParameters=[1 0 0 0 0]  TsPowergui=0  TsBlock=-1  IterativeModel=Trapezoidal non iterative  IterativeDiscreteModel=Trapezoidal non iterative  BusType=PV  Pref=0  Qref=0  Qmin=-inf  Qmax=inf  PLF=0  QLF=0
  Universal Bridge : spsUniversalBridgeLib/Universal Bridge  Arms=3  SnubberResistance=2*Ts_snub/(Pnom/(1000*2*pi*Fnom*Vnom_gen^2))  SnubberCapacitance=Pnom/(1000*2*pi*Fnom*Vnom_gen^2)  Device=Diodes  Ron=1e-6/Nb_wt  Lon=0  ForwardVoltages="[  0  0  ]"  ForwardVoltage=0  GTOparameters=[ 10e-6 , 20e-6 ]  IGBTparameters=[ 1e-6 , 2e-6 ]  Measurements=None  Measurements_2=None  converterType=Rectifier
  Universal Bridge1 : spsUniversalBridgeLib/Universal Bridge  Arms=3  SnubberResistance=1e6/Nb_wt  SnubberCapacitance=inf  Device=IGBT / Diodes  Ron=1e-6/Nb_wt  Lon=0  ForwardVoltages="[  0  0  ]"  ForwardVoltage=0  GTOparameters=[ 10e-6 , 20e-6 ]  IGBTparameters=[ 1e-6 , 2e-6 ]*0  Measurements=None  Measurements_2=None  converterType=Rectifier
  Wind Turbine : Subsystem  mask(Wind Turbine){Prated=Pmec, c1_c8=c1_c8, K1_K2=K1_K2, wind0=wind0, Ts=Ts}
      mask prompts: Prated "Nominal mechanical output power (W):"; c1_c8 "Coefficients [c1 ... c8]"; K1_K2 "Parameters [K1 K2]"; wind0 "Initial wind speed (m/s):"; Ts "Sample time (s):"
      mask help:
      | This block implements a generic wind turbine models.
      |
      | The first input is the turbine speed in per unit of the generator base speed. For a synchronous or asynchronous generator, the base speed is the synchronous speed. For a permanent-magnet generator, the base speed is defined as the speed producing nominal voltage at  no load. The second input is the blade pitch angle in degrees. The third input is the wind speed in m/s.
      |
      | The output is the torque applied to the drive train in per unit based on the nominal power of the turbine and the base speed of the generator.
      mask init:
      | c1 = c1_c8(1);
      | c2 = c1_c8(2);
      | c3 = c1_c8(3);
      | c4 = c1_c8(4);
      | c5 = c1_c8(5);
      | c6 = c1_c8(6);
      | c7 = c1_c8(7);;
      | c8 = c1_c8(8);
      | 
      | K1=K1_K2(1);
      | K2=K1_K2(2);
      settings: OpenFcn=power_openblockproxy();
      mask Display: disp('');
  deg->rd : Gain  Gain=pi/180  SaturateOnIntegerOverflow=on  OutDataTypeStr=Inherit: Same as input  ParamDataTypeStr=Inherit: Same as input
  A : PMIOPort  Tag=PMCPort  Side=Left
  B : PMIOPort  Tag=PMCPort  Port=2  Side=Left
  C : PMIOPort  Tag=PMCPort  Port=3  Side=Left
  m : Outport
  wires:
  [Vf] -> Synchronous Machine pu Standard/2
  Wind Turbine/1(Tt (pu)) -> Drive Train/1(T_wt (pu))
  [wr] -> Drive Train/2(Generator speed (pu))
  Drive Train/2(T_shaft (pu)) -> Power base for the Generator/1
  Power base for the Generator/1 -> [Tm]
  "Wind (m/s) "/1 -> Wind Turbine/3(Wind speed (m/s))
  Drive Train/1(W_wt (pu)) -> Wind Turbine/1(W_wt (pu))
  [Pitch] -> Wind Turbine/2(Pitch angle (deg))
  Bus Selector/2 -> deg->rd/1  "<Rotor mechanical angle  theta (deg)>"
  deg->rd/1 -> [angle_rotor]
  Bus Selector/1 -> [wr]  "<Rotor speed  wm  (pu)>"
  [wr] -> Product/1
  Synchronous Machine pu Standard/1 -> Bus Selector/1
  B_grid_conv/1 -> [Vabc_grid_conv]
  [Tm] -> Product/2
  Product/1 -> Synchronous Machine pu Standard/1, [Pm_gen]
  B_grid/1 -> [Vabc_grid]
  B_grid/2 -> [Iabc_grid_conv]
  B_gen/1 -> [Vabc_LL_stator]
  B_gen/2 -> [Iabc_stator]
  [Vabc_grid] -> Control/1(Vabc_grid)
  [Iabc_grid_conv] -> Control/2(Iabc_grid_conv)
  [Vabc_LL_stator] -> Control/3(Vabc_LL_stator)
  [Iabc_stator] -> Control/4(Iabc_stator)
  [Vdc] -> Control/6(Vdc)
  Qref_pu/1 -> Control/7(Qref)
  [angle_rotor] -> Control/8(angle_rotor)
  [wr] -> Control/9(wr)
  Control/1(Inverter_Pulses) -> [Inverter_Pulses]
  Control/2(Boost_Pulse) -> [Boost_Pulse]
  Control/3(Pitch_angle) -> [Pitch]
  Control/4(Vf) -> [Vf]
  [Inverter_Pulses] -> Universal Bridge1/1
  [Boost_Pulse] -> Ideal Switch/1
  Control/5(PQ_pu) -> [PQ_pu]
  [Vabc_LL_stator] -> Bus Creator/1  "Vabc_stator_pu"
  [Iabc_stator] -> Bus Creator/2  "Iabc_stator_pu"
  [Vabc_grid] -> Bus Creator/3  "Vabc_grid_pu"
  Bus Creator/1 -> m/1
  [Vabc_grid_conv] -> Bus Creator/4  "Vabc_grid_conv_pu"
  [Iabc_grid_conv] -> Bus Creator/5  "Iabc_grid_conv_pu"
  [Vf] -> Bus Creator/6  "Vfield_pu"
  [wr] -> Bus Creator/7  "wr_pu"
  [Pm_gen] -> Bus Creator/8  "Pm_gen_pu"
  [Pitch] -> Bus Creator/9  "Pitch_deg"
  [Vdc] -> Bus Creator/10  "Vdc_V"
  [PQ_pu] -> Bus Creator/11  "PQ_pu"
  [IL] -> Control/5(IL)
  connections:
  B_grid/RConn1 -- "Choke "/LConn1
  B_grid/RConn2 -- "Choke "/LConn2
  B_grid/RConn3 -- "Choke "/LConn3
  A/RConn1 -- B_grid/LConn1 -- Filter Q=50/LConn1
  Filter Q=50/LConn2 -- B_grid/LConn2 -- B/RConn1
  Filter Q=50/LConn3 -- B_grid/LConn3 -- C/RConn1
  "Choke "/RConn1 -- B_grid_conv/LConn1
  "Choke "/RConn2 -- B_grid_conv/LConn2
  "Choke "/RConn3 -- B_grid_conv/LConn3
  Series RLC Branch1/LConn1 -- Universal Bridge/RConn1
  Universal Bridge/LConn1 -- B_gen/LConn1
  Universal Bridge/LConn2 -- B_gen/LConn2
  Universal Bridge/LConn3 -- B_gen/LConn3
  Diode/LConn1 -- Series RLC Branch1/RConn1 -- Ideal Switch/LConn1
  Universal Bridge1/LConn1 -- B_grid_conv/RConn1
  Universal Bridge1/LConn2 -- B_grid_conv/RConn2
  Universal Bridge1/LConn3 -- B_grid_conv/RConn3
  Universal Bridge1/RConn1 -- Diode/RConn1 -- C_DClink/LConn1
  Universal Bridge/RConn2 -- Universal Bridge1/RConn2 -- C_DClink/RConn1 -- Ideal Switch/RConn1
  Synchronous Machine pu Standard/RConn3 -- B_gen/RConn3
  Synchronous Machine pu Standard/RConn2 -- B_gen/RConn2
  Synchronous Machine pu Standard/RConn1 -- B_gen/RConn1

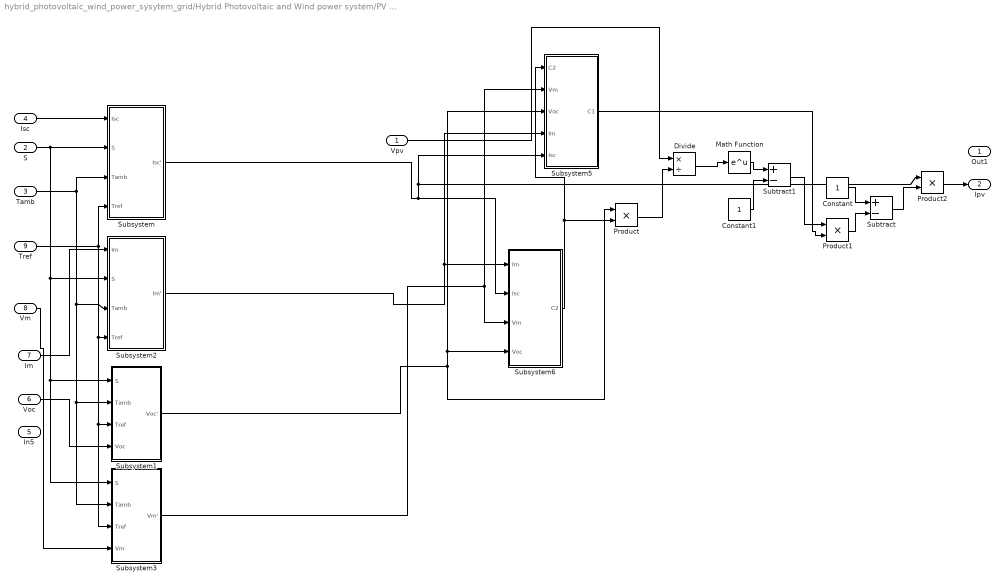
== system hybrid_photovoltaic_wind_power_sysytem_grid/Hybrid Photovoltaic and Wind power system/PV array1/Subsystem1 ==
  Vpv : Inport
  S : Inport  Port=2
  Tamb : Inport  Port=3
  Isc : Inport  Port=4
  In5 : Inport  Port=5
  Voc : Inport  Port=6
  Im : Inport  Port=7
  Vm : Inport  Port=8
  Tref : Inport  Port=9
  Constant : Constant
  Constant1 : Constant
  Divide : Product  Inputs=*/
  Math Function : Math  SignedPower=on
  Product : Product  RndMeth=Zero
  Product1 : Product  RndMeth=Zero
  Product2 : Product  RndMeth=Zero
  Subsystem : Subsystem
  Subsystem1 : Subsystem
  Subsystem2 : Subsystem
  Subsystem3 : Subsystem
  Subsystem5 : Subsystem
  Subsystem6 : Subsystem
  Subtract : Sum  Inputs=+-
  Subtract1 : Sum  Inputs=+-
  Out1 : Outport
  Ipv : Outport  Port=2
  wires:
  Vm/1 -> Subsystem3/4(Vm)
  Voc/1 -> Subsystem1/4(Voc)
  Im/1 -> Subsystem2/1(Im)
  Tref/1 -> Subsystem/4(Tref), Subsystem2/4(Tref), Subsystem3/3(Tref), Subsystem1/3(Tref)
  Tamb/1 -> Subsystem/3(Tamb), Subsystem2/3(Tamb), Subsystem3/2(Tamb), Subsystem1/2(Tamb)
  S/1 -> Subsystem/2(S), Subsystem2/2(S), Subsystem3/1(S), Subsystem1/1(S)
  Isc/1 -> Subsystem/1(Isc)
  Subsystem5/1(C1) -> Product1/2
  Vpv/1 -> Divide/1
  Subsystem6/1(C2) -> Product/2, Subsystem5/1(C2)
  Subsystem3/1(Vm') -> Subsystem6/3(Vm), Subsystem5/2(Vm)
  Subsystem1/1(Voc') -> Subsystem6/4(Voc), Subsystem5/3(Voc), Product/1
  Subsystem/1(Isc') -> Subsystem5/5(Isc), Product2/1, Subsystem6/2(Isc)
  Subsystem2/1(Im') -> Subsystem5/4(Im), Subsystem6/1(Im)
  Subtract1/1 -> Product1/1
  Constant1/1 -> Subtract1/2
  Math Function/1 -> Subtract1/1
  Divide/1 -> Math Function/1
  Product2/1 -> Ipv/1
  Subtract/1 -> Product2/2
  Product1/1 -> Subtract/2
  Constant/1 -> Subtract/1
  Product/1 -> Divide/2
